simulink library "Weather2WDB"  (Simulink 7.6)
settings: Solver=ode45  StartTime=0.0  StopTime=10.0  RelTol=1e-3
libraries: carnot x1
settings Model: Creator=lena.frank  LastModifiedBy=drhf

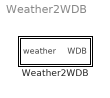
== system Weather2WDB ==
  Weather2WDB : Subsystem
      mask Type: weather 2 WDB
      mask Description:
      | Creates the weather data bus WDB from the weather data vector.
      | Format in weather data vector:
      | 1  timevalue (comment line) format YYYYMMDDHHMM    -
      | 2  zenith angle of sun (at time, not averaged)       degree
      | 3  azimuth angle of sun (0°=south, east negative) degree
      | 4  beam solar radiation on a normal surface         W/m^2
      | 5  diffuse solar radiation on a horizontal surface   W/m^2
      | 6  ambient temperature                                    degree celsius
      | 7  radiation temperature of sky                          degree celsius
      | 8  relative humidity                                           percent
      | 9  precipitation                                                 m/s
      | 10 cloud index (0=no cloud, 1=covered sky)         -
      | 11 station pressure                                           Pa
      | 12 mean wind speed                                         m/s
      | 13 wind direction (north=0° west=270°)             degree
      | 14 incidence angle on surface (0° = vertical)      degree
      | 15 longitudinal incidence angle                       degree
      | 16 transversal incidence angle                        degree
      | 17 direct solar radiation on surface                 W/m²
      | 18 diffuse solar radiation on surface                W/m²

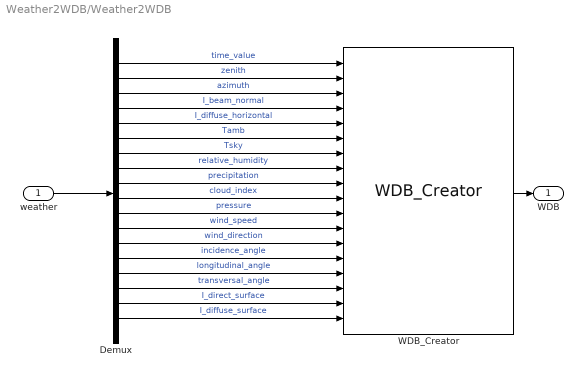
== system Weather2WDB/Weather2WDB ==
  weather : Inport
  Demux : Demux  Outputs=18
  WDB_Creator : carnot/Basic/Weather_and_Sun/WDB_Creator  SystemSampleTime=-1
  WDB : Outport
  wires:
  Demux/18 -> WDB_Creator/18  "I_diffuse_surface"
  Demux/17 -> WDB_Creator/17  "I_direct_surface"
  Demux/16 -> WDB_Creator/16  "transversal_angle"
  Demux/15 -> WDB_Creator/15  "longitudinal_angle"
  Demux/14 -> WDB_Creator/14  "incidence_angle"
  Demux/13 -> WDB_Creator/13  "wind_direction"
  Demux/12 -> WDB_Creator/12  "wind_speed"
  Demux/11 -> WDB_Creator/11  "pressure"
  Demux/10 -> WDB_Creator/10  "cloud_index"
  Demux/9 -> WDB_Creator/9  "precipitation"
  Demux/8 -> WDB_Creator/8  "relative_humidity"
  Demux/7 -> WDB_Creator/7  "Tsky"
  Demux/6 -> WDB_Creator/6  "Tamb"
  Demux/5 -> WDB_Creator/5  "I_diffuse_horizontal"
  Demux/4 -> WDB_Creator/4  "I_beam_normal"
  Demux/3 -> WDB_Creator/3  "azimuth"
  Demux/2 -> WDB_Creator/2  "zenith"
  Demux/1 -> WDB_Creator/1  "time_value"
  WDB_Creator/1 -> WDB/1
  weather/1 -> Demux/1
